simulink model "MultirotorSimFSFBTranslationOnly"  (R2018b)
settings: Solver=VariableStepAuto  StartTime=0.0  StopTime=Simulation.T_END  MaxStep=Simulation.TS_MAX  RelTol=1e-3  EnableMultiTasking=on
PreLoadFcn:
  | % InitializeParameters;
undefined symbols (not defined in the file): Aero, Initial, K, Uav, Wind
libraries: QuaternionLibrary x12
settings Model: Creator=jban039  LastModifiedBy=jban039
settings DataIOCC: Decimation=10  ExternalInput=getinputstruct(op)  InitialState=getstatestruct(op)  SaveFormat=StructureWithTime  SignalLogging=off  ReturnWorkspaceOutputs=on  OutputTimes=Simulation.T_OUT
settings OptimizationCC: LifeSpan=inf
settings DebuggingCC: ReadBeforeWriteMsg=DisableAll  WriteAfterWriteMsg=DisableAll  WriteAfterReadMsg=DisableAll  MultiTaskDSMMsg=none  UnconnectedLineMsg=none  AllowSymbolicDim=off  SFUnexpectedBacktrackingDiag=warning  SFNoUnconditionalDefaultTransitionDiag=warning  SFExecutionAtInitializationDiag=none
settings ModelReferenceCC: UpdateModelReferenceTargets=IfOutOfDate  ModelReferenceMinAlgLoopOccurrences=on  PropagateSignalLabelsOutOfModel=off
settings SFSimCC: SFSimEcho=off  SimUseLocalCustomCode=off
settings RTWCC: RTWUseLocalCustomCode=off
settings CodeAppCC: StateflowObjectComments=on
settings GRTTargetCC: TargetLangStandard=C89/C90 (ANSI)
settings ConfigComp: CovMetricSettings=dw  CovHtmlReporting=on  CovSaveCumulativeToWorkspaceVar=on  CovSaveSingleToWorkspaceVar=on  CovExternalEMLEnable=off

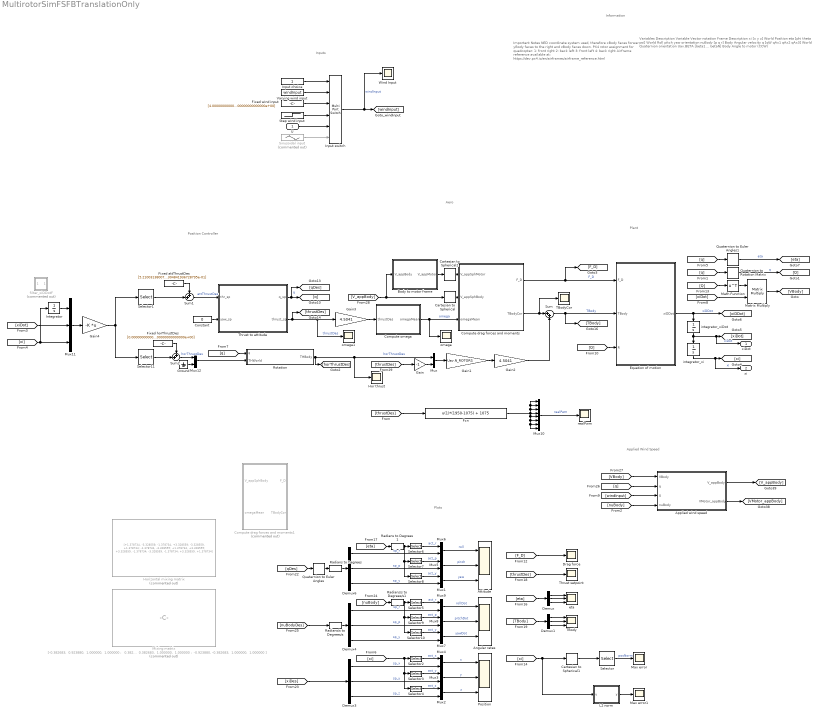
== system MultirotorSimFSFBTranslationOnly ==
  note: Plots
  note: Inputs
  note: Plant
  note: Position Controller
  note: Applied Wind Speed
  note: Important Notes
      |
      | NED coordinate system used, therefore xBody faces forward, yBody faces to the right and zBody faces down.
      | PX4 rotor assignment for quadcopter:
      | 1: front right
      | 2: back left
      | 3: front left
      | 4: back right
      | Airframe reference available at:
      | https://dev.px4.io/en/airframes/airframe_reference.html
  note: Variables Description
      |
      | Variable
      | Vector notation
      | Frame
      | Description
      |
      | xi
      | [x y z]
      | World
      | Position
      |
      | eta
      | [phi theta psi]
      | World
      | Roll pitch yaw orientation
      |
      | nuBody
      | [p q r]
      | Body
      | Angular velocity
      |
      | q
      | [qW qAx1 qAx2 qAx3]
      | World
      | Quaternion orientation
      |
      | Uav.BETA
      | [beta1 ... betaN]
      | Body
      | Angle to motor (CCW)
  note: Information
  note: Aero
  U : Inport  PortDimensions=3
  Angular rates : Scope  NumInputPorts=3
  Applied wind speed : Subsystem
  Attitude : Scope  NumInputPorts=3
  Body to motor frame : MATLAB Function  TreatAsAtomicUnit=on
  Cartesian to Spherical : QuaternionLibrary/Cartesian to Spherical
  Cartesian to Spherical1 : QuaternionLibrary/Cartesian to Spherical
  Cartesian to Spherical2 : QuaternionLibrary/Cartesian to Spherical
  Compute drag forces and moments : MATLAB Function  TreatAsAtomicUnit=on
  Compute drag forces and moments1 : MATLAB Function  Commented=on  TreatAsAtomicUnit=on
  Compute omega : MATLAB Function  TreatAsAtomicUnit=on
  Constant : Constant  Value=0
  Demux{,1,3..4,6} (5 alike) : Demux  Outputs=3
  Drag force : Scope
  Equation of motion : MATLAB Function  TreatAsAtomicUnit=on
  Fcn : Fcn  Expr=u(1)*(1950-1075) + 1075
  Fixed attThrustDes : Constant  Value=[5.210031380070558e-02;0.000000000000000e+00;-5.304841936728795e-01]
  Fixed horThrustDes : Constant  Value=[0.000000000000000e+00;0.000000000000000e+00]
  Fixed wind input : Constant  Value=[4.000000000000000e+00;0.000000000000000e+00;0.000000000000000e+00]
  Gain : Gain  Gain=-1
  Gain1 : Gain  Gain=Uav.N_ROTORS
  Gain2 : Gain  Gain=4.5041
  Gain3 : Gain  Gain=4.5041
  Gain4 : Gain  Gain=-K  Multiplication=Matrix(K*u)
  Ground : Ground
  Hor thrust : Scope
  Horizontal mixing matrix : Constant  Commented=on  Value=|
      | [+1.378734, -3.328559;
      |  -1.378734, +3.328559;
      |  -3.328559, +1.378734;
      |  -1.378734, -3.328559;
      |  +1.378734, +3.328559;
      |  +3.328559, -1.378734;
      |  -3.328559, -1.378734;
      |  +3.328559, +1.378734]
  Input choice : Constant
  Input switch : MultiPortSwitch  Inputs=5
  Integrator : Integrator
  L2 norm : MATLAB Function  TreatAsAtomicUnit=on
  Math Function : Math  Operator=transpose  SaturateOnIntegerOverflow=on
  Matrix Multiply : Product  Multiplication=Matrix(*)
  Max error : Scope
  Max error1 : Scope
  Mixing matrix : Constant  Commented=on  Value=|
      | [-0.382683,  0.923880,  1.000000,  1.000000 ;
      |   0.382683, -0.923880,  1.000000,  1.000000 ;
      |  -0.923880,  0.382683, -1.000000,  1.000000 ;
      |  -0.382683, -0.923880, -1.000000,  1.000000 ;
      |   0.382683,  0.923880, -1.000000,  1.000000 ;
      |   0.923880, -0.382683, -1.000000,  1.000000 ;
      |   0.923880,  0.382683,  1.000000,  1.000000 ;
      |  -0.923880, -0.382683,  1.000000,  1.000000 ]
  Mux{,1..9,12} (11 alike) : Mux  Inputs=2
  Mux10 : Mux  Inputs=8
  Mux11 : Mux  Inputs=3
  Position : Scope  NumInputPorts=3
  Quaternion to Euler Angles : QuaternionLibrary/Quaternion to Euler Angles
  Quaternion to Euler Angles1 : QuaternionLibrary/Quaternion to Euler Angles
  Quaternion to Rotation Matrix : QuaternionLibrary/Quaternion to Rotation Matrix
  "Radians to Degrees " : QuaternionLibrary/Radians to Degrees   SystemSampleTime=-1
  Radians to Degrees 1 : QuaternionLibrary/Radians to Degrees   SystemSampleTime=-1
  Radians/s to Degrees/s : QuaternionLibrary/Radians//s to Degrees//s  SystemSampleTime=-1
  Radians/s to Degrees/s1 : QuaternionLibrary/Radians//s to Degrees//s  SystemSampleTime=-1
  Rotation : Subsystem
  Selector : Selector  InputPortWidth=3  IndexOptions=Index vector (dialog)  Indices=[3]  OutputSizes=1
  Selector1 : Selector  InputPortWidth=5  IndexOptions=Index vector (dialog)  Indices=[3:5]  OutputSizes=1
  Selector10 : Selector  InputPortWidth=3  IndexOptions=Index vector (dialog)  Indices=3  OutputSizes=1
  Selector11 : Selector  InputPortWidth=5  IndexOptions=Index vector (dialog)  Indices=[1 2]  OutputSizes=1
  Selector2 : Selector  InputPortWidth=3  IndexOptions=Index vector (dialog)  Indices=1  OutputSizes=1
  Selector3 : Selector  InputPortWidth=3  IndexOptions=Index vector (dialog)  Indices=2  OutputSizes=1
  Selector4 : Selector  InputPortWidth=3  IndexOptions=Index vector (dialog)  Indices=3  OutputSizes=1
  Selector5 : Selector  InputPortWidth=3  IndexOptions=Index vector (dialog)  Indices=1  OutputSizes=1
  Selector6 : Selector  InputPortWidth=3  IndexOptions=Index vector (dialog)  Indices=1  OutputSizes=1
  Selector7 : Selector  InputPortWidth=3  IndexOptions=Index vector (dialog)  Indices=2  OutputSizes=1
  Selector8 : Selector  InputPortWidth=3  IndexOptions=Index vector (dialog)  Indices=3  OutputSizes=1
  Selector9 : Selector  InputPortWidth=3  IndexOptions=Index vector (dialog)  Indices=2  OutputSizes=1
  Sinusoidal input : Sin  Commented=on  Amplitude=Wind.Ampl  Bias=Wind.Bias  Frequency=Wind.Freq  SampleTime=0
  Step wind input : Step  Time=Wind.StepTime  Before=Wind.StepInit  After=Wind.StepFinal  SampleTime=0
  Sum : Sum  Inputs=|++
  Sum1 : Sum  Inputs=++|
  Sum2 : Sum  Inputs=++|
  TBody : Scope  NumInputPorts=3
  TBodyCor : Scope
  Thrust setpoint : Scope
  Thrust to attitude : MATLAB Function  TreatAsAtomicUnit=on
  Varying wind input : FromWorkspace  VariableName=windInput  SampleTime=0
  Wind Input : Scope
  eta : Scope  NumInputPorts=3
  filter_xiDDotF : Subsystem  Commented=on  mask{PID_FC=5}
      mask prompts: PID_FC "D filter cutoff"
      mask Display: disp('s')
  integrator_xi : Integrator  InitialCondition=Initial.XI  ContinuousStateAttributes='xi'
  integrator_xiDot : Integrator  InitialCondition=Initial.XI_DOT  ContinuousStateAttributes='xiDot'
  omega : Scope
  omega1 : Scope
  realPwm : Scope
  xiDot : Outport
  xi : Outport  Port=2
  wires:
  Sum/1 -> Equation of motion/2(TBody), [TBody]  "TBody"
  Matrix Multiply/1 -> [VBody]
  integrator_xi/1 -> xi/1, [xi]  "xi"
  integrator_xiDot/1 -> xiDot/1, [xiDot], integrator_xi/1  "xiDot"
  Equation of motion/1(xiDDot) -> [xiDDot], integrator_xiDot/1  "xiDDot"
  Quaternion to Euler Angles1/1 -> [eta]  "eta"
  Thrust to attitude/1(q_sp) -> [q], [qDes]  "q"
  [VBody] -> Applied wind speed/1(VBody)
  [q] -> Applied wind speed/2(q)
  [windInput] -> Applied wind speed/3(U)
  Applied wind speed/1(V_appBody) -> [V_appBody]
  Applied wind speed/2(VMotor_appBody) -> [VMotor_appBody]
  [nuBody] -> Applied wind speed/4(nuBody)
  Mux7/1 -> Angular rates/3  "yawDot"
  [nuBody] -> Radians/s to Degrees/s1/1
  Radians/s to Degrees/s1/1 -> Selector5/1, Selector9/1, Selector10/1
  Radians/s to Degrees/s/1 -> Demux4/1
  Mux8/1 -> Angular rates/2  "pitchDot"
  Mux9/1 -> Angular rates/1  "rollDot"
  Selector10/1 -> Mux7/1  "act_y"
  Demux4/2 -> Mux8/2  "sp_p"
  Demux4/1 -> Mux9/2  "sp_r"
  [nuBodyDes] -> Radians/s to Degrees/s/1
  Selector9/1 -> Mux8/1  "act_p"
  Selector5/1 -> Mux9/1  "act_r"
  Demux4/3 -> Mux7/2  "sp_y"
  Mux2/1 -> Position/3  "z"
  [xi] -> Selector2/1, Selector3/1, Selector4/1
  [xiDes] -> Demux3/1
  Mux3/1 -> Position/2  "y"
  Mux4/1 -> Position/1  "x"
  Selector4/1 -> Mux2/1  "act_z"
  Demux3/2 -> Mux3/2  "sp_y"
  Demux3/1 -> Mux4/2  "sp_x"
  Selector3/1 -> Mux3/1  "act_y"
  Selector2/1 -> Mux4/1  "act_x"
  Demux3/3 -> Mux2/2  "sp_z"
  L2 norm/1(y) -> Max error1/1
  [F_D] -> Drag force/1
  Selector/1 -> Max error/1  "posNorm"
  Demux1/1 -> TBody/1
  [TBody] -> Demux1/1
  Demux1/2 -> TBody/2
  Demux1/3 -> TBody/3
  [thrustDes] -> Thrust setpoint/1
  Demux6/3 -> Mux1/2  "sp_y"
  Selector6/1 -> Mux6/1  "act_r"
  Selector7/1 -> Mux5/1  "act_p"
  Quaternion to Euler Angles/1 -> "Radians to Degrees "/1
  Demux6/1 -> Mux6/2  "sp_r"
  Demux6/2 -> Mux5/2  "sp_p"
  Selector8/1 -> Mux1/1  "act_y"
  [qDes] -> Quaternion to Euler Angles/1
  Mux6/1 -> Attitude/1  "roll"
  Mux5/1 -> Attitude/2  "pitch"
  "Radians to Degrees "/1 -> Demux6/1
  Radians to Degrees 1/1 -> Selector8/1, Selector7/1, Selector6/1
  [eta] -> Radians to Degrees 1/1
  Mux1/1 -> Attitude/3  "yaw"
  Demux/3 -> eta/3
  Demux/2 -> eta/2
  Demux/1 -> eta/1
  [eta] -> Demux/1
  [xi] -> Cartesian to Spherical1/1, L2 norm/1(u)
  Sinusoidal input/1 -> Input switch/6
  U/1 -> Input switch/5
  Input choice/1 -> Input switch/1
  Step wind input/1 -> Input switch/4
  Input switch/1 -> [windInput], Wind Input/1  "windInput"
  Fixed wind input/1 -> Input switch/3
  Varying wind input/1 -> Input switch/2
  [Q] -> Equation of motion/3(R)
  [q] -> Quaternion to Euler Angles1/1
  [q] -> Quaternion to Rotation Matrix/1
  Quaternion to Rotation Matrix/1 -> [Q]  "q"
  Math Function/1 -> Matrix Multiply/1
  [xiDot] -> Matrix Multiply/2
  [Q] -> Math Function/1
  [V_appBody] -> Cartesian to Spherical/1, Body to motor frame/1(V_appBody)
  Cartesian to Spherical/1 -> Compute drag forces and moments/2(V_appSphBody)
  Compute omega/1(omegaMean) -> Compute drag forces and moments/3(omegaMean), omega/1  "omega"
  Rotation/1(THBody) -> [horThrustDes], Mux/1, Hor thrust/1  "horThrustDes"
  [thrustDes] -> Gain/1
  Compute drag forces and moments/1(F_D) -> [F_D], Equation of motion/1(F_D)  "F_D"
  Compute drag forces and moments/2(TBodyCor) -> TBodyCor/1, Sum/1
  Mux/1 -> Gain1/1
  Gain/1 -> Mux/2
  Gain2/1 -> Sum/2
  Gain3/1 -> Compute omega/1(thrustDes)
  [thrustDes] -> Fcn/1
  Mux10/1 -> realPwm/1  "realPwm"
  Fcn/1 -> Mux10/8, Mux10/7, Mux10/6, Mux10/5, Mux10/1, Mux10/2, Mux10/3, Mux10/4
  Thrust to attitude/2(thrust_sp) -> omega1/1, Gain3/1, [thrustDes]  "thrustDes"
  Fixed horThrustDes/1 -> Sum2/1
  Cartesian to Spherical1/1 -> Selector/1
  Gain1/1 -> Gain2/1
  Body to motor frame/1(V_appMotor) -> Cartesian to Spherical2/1
  Cartesian to Spherical2/1 -> Compute drag forces and moments/1(V_appSphMotor)
  Constant/1 -> Thrust to attitude/2(yaw_sp)
  Sum1/1 -> Thrust to attitude/1(thr_sp)  "attThrustDes"
  Fixed attThrustDes/1 -> Sum1/1
  Selector1/1 -> Sum1/2
  Selector11/1 -> Sum2/2
  [xiDot] -> Mux11/2
  [xi] -> Mux11/3, Integrator/1
  Mux11/1 -> Gain4/1
  Gain4/1 -> Selector1/1, Selector11/1
  Integrator/1 -> Mux11/1
  Sum2/1 -> Mux12/1  "horThrustDes"
  Ground/1 -> Mux12/2
  Mux12/1 -> Rotation/2(THWorld)
  [q] -> Rotation/1(q)

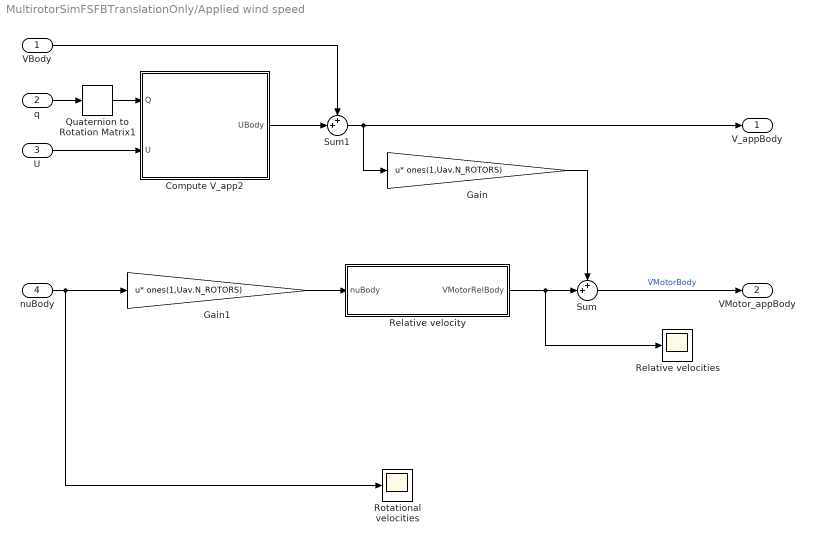
== system MultirotorSimFSFBTranslationOnly/Applied wind speed ==
  VBody : Inport  Unit=m/s
  q : Inport  Port=2
  U : Inport  Port=3  Unit=m/s
  nuBody : Inport  Port=4  Unit=rad/s
  Compute V_app2 : MATLAB Function  TreatAsAtomicUnit=on
  Gain : Gain  Gain=ones(1,Uav.N_ROTORS)  Multiplication=Matrix(u*K)
  Gain1 : Gain  Gain=ones(1,Uav.N_ROTORS)  Multiplication=Matrix(u*K)
  Quaternion to Rotation Matrix1 : QuaternionLibrary/Quaternion to Rotation Matrix
  Relative velocities : Scope
  Relative velocity : MATLAB Function  TreatAsAtomicUnit=on
  Rotational velocities : Scope
  Sum : Sum  Inputs=++|
  Sum1 : Sum  Inputs=++|
  V_appBody : Outport  Unit=m/s
  VMotor_appBody : Outport  Port=2  Unit=m/s  PortDimensions=[3,Uav.N_ROTORS]
  wires:
  U/1 -> Compute V_app2/2(U)
  Sum/1 -> VMotor_appBody/1  "VMotorBody"
  Quaternion to Rotation Matrix1/1 -> Compute V_app2/1(Q)
  nuBody/1 -> Gain1/1, Rotational velocities/1
  Gain/1 -> Sum/1
  VBody/1 -> Sum1/1
  q/1 -> Quaternion to Rotation Matrix1/1
  Relative velocity/1(VMotorRelBody) -> Relative velocities/1, Sum/2
  Compute V_app2/1(UBody) -> Sum1/2
  Sum1/1 -> Gain/1, V_appBody/1
  Gain1/1 -> Relative velocity/1(nuBody)

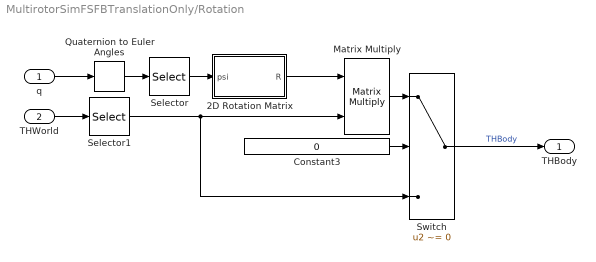
== system MultirotorSimFSFBTranslationOnly/Rotation ==
  q : Inport
  THWorld : Inport  Port=2
  2D Rotation Matrix : Subsystem
  Constant3 : Constant  Value=0
  Matrix Multiply : Product  Multiplication=Matrix(*)
  Quaternion to Euler Angles : QuaternionLibrary/Quaternion to Euler Angles
  Selector : Selector  InputPortWidth=3  IndexOptions=Index vector (dialog)  Indices=3  OutputSizes=1
  Selector1 : Selector  InputPortWidth=3  IndexOptions=Index vector (dialog)  Indices=[1 2]  OutputSizes=1
  Switch : Switch  Criteria=u2 ~= 0
  THBody : Outport
  wires:
  Selector1/1 -> Matrix Multiply/2, Switch/3
  Constant3/1 -> Switch/2
  Selector/1 -> 2D Rotation Matrix/1(psi)
  Quaternion to Euler Angles/1 -> Selector/1
  2D Rotation Matrix/1(R) -> Matrix Multiply/1
  Switch/1 -> THBody/1  "THBody"
  Matrix Multiply/1 -> Switch/1
  THWorld/1 -> Selector1/1
  q/1 -> Quaternion to Euler Angles/1

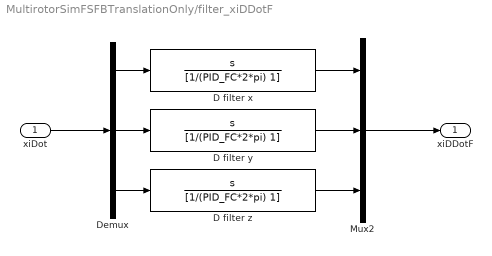
== system MultirotorSimFSFBTranslationOnly/filter_xiDDotF ==
  xiDot : Inport  Unit=m/s
  D filter x : TransferFcn  Numerator=[1 0]  Denominator=[1/(PID_FC*2*pi) 1]  ContinuousStateAttributes='velPID_D_x'
  D filter y : TransferFcn  Numerator=[1 0]  Denominator=[1/(PID_FC*2*pi) 1]  ContinuousStateAttributes='velPID_D_y'
  D filter z : TransferFcn  Numerator=[1 0]  Denominator=[1/(PID_FC*2*pi) 1]  ContinuousStateAttributes='velPID_D_z'
  Demux : Demux  Outputs=3
  Mux2 : Mux  Inputs=3
  xiDDotF : Outport  Unit=m/s^2
  wires:
  Mux2/1 -> xiDDotF/1
  Demux/3 -> D filter z/1
  Demux/1 -> D filter x/1
  D filter z/1 -> Mux2/3
  xiDot/1 -> Demux/1
  D filter y/1 -> Mux2/2
  Demux/2 -> D filter y/1
  D filter x/1 -> Mux2/1

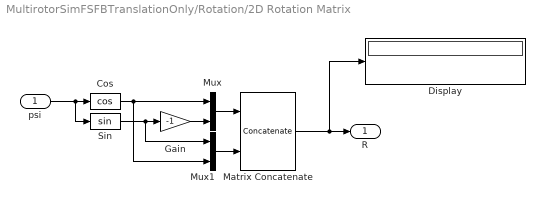
== system MultirotorSimFSFBTranslationOnly/Rotation/2D Rotation Matrix ==
  psi : Inport
  Cos : Trigonometry  Operator=cos
  Display : Display
  Gain : Gain  Gain=-1
  Matrix Concatenate : Concatenate  Mode=Multidimensional array  ConcatenateDimension=2
  Mux : Mux  Inputs=2
  Mux1 : Mux  Inputs=2
  Sin : Trigonometry
  R : Outport
  wires:
  psi/1 -> Cos/1, Sin/1
  Matrix Concatenate/1 -> R/1, Display/1
  Mux1/1 -> Matrix Concatenate/2
  Gain/1 -> Mux/2
  Mux/1 -> Matrix Concatenate/1
  Sin/1 -> Gain/1, Mux1/1
  Cos/1 -> Mux/1, Mux1/2

== matlab function MultirotorSimFSFBTranslationOnly/Body to motor frame ==
  data: V_appBody input; V_appMotor output; Uav parameter
function V_appMotor = BodyToMotor( V_appBody, Uav )
%#codegen
    V_appMotor = [Uav.GAMMA';Uav.GAMMA';Uav.GAMMA'] .* 0;
    for i = 1:Uav.N_ROTORS
        V_appMotor(:,i) = Uav.R_MOTOR_TO_BODY(:,:,i)' * V_appBody;
    end
end

== matlab function MultirotorSimFSFBTranslationOnly/Compute omega ==
  data: thrustDes input; omegaMean output; Uav parameter; Aero parameter
function omegaMean = CalcOmega( thrustDes, Uav, Aero)
%#codegen
    thrustDesMotor = thrustDes ./ cos(Uav.ZETA);
    Cz2 = dot( Aero.Cz2.coefs, [0, 1]);
    omegaMean = sqrt( thrustDesMotor .* 2 ./ ( Uav.RHO_AIR .* Cz2 .* Uav.D_PROP^2 .* Uav.A_PROP ) );
end

== matlab function MultirotorSimFSFBTranslationOnly/Compute drag forces and moments1 ==
  data: V_appSphBody input; omegaMean input; F_D output; Uav parameter; Aero parameter; TBodyCor output
function [F_D, TBodyCor] = ComputeAero( V_appSphBody, omegaMean, Uav, Aero )
%#codegen
    % Body aerodynamic forces
    beta  = V_appSphBody(1);
    alpha = V_appSphBody(2);
    U     = V_appSphBody(3);

    Cz1 = dot( Aero.Cz1.coefs, [sin(alpha), 1] );
    Cx1 = dot( Aero.Cx1.coefs, [cos(alpha), cos(3*alpha), cos(7*alpha)] );
    faero_z = -0.5 .* Uav.RHO_AIR .* U^2 .* Cz1 * Uav.A_UAV;
    faero_x = -0.5 .* Uav.RHO_AIR .* U^2 .* Cx1 * Uav.A_UAV;
    F_D = [faero_x*cos(beta); faero_x*sin(beta); faero_z];

    % Rotor aerodynamic forces
    lambda = omegaMean * Uav.D_PROP / ( 2 * U );
    p = Aero.Cx2.coefs;
    Cx2 = p(1) * ( 1 - exp(-p(2).*lambda) ) .* cos(alpha) + ...
          p(3) * ( 1 - exp(-p(4).*lambda) ) .* cos(3*alpha);
    Tx    = -0.5 .* Uav.RHO_AIR .* (Cx2)' .* U .* omegaMean' .* Uav.D_PROP .* Uav.A_PROP;
    TBodyHor = [ Tx.*cos(beta); Tx.*sin(beta); 0 ] .* Uav.N_ROTORS;
    
    TBodyIndividual   = zeros(3,Uav.N_ROTORS);
    for i = 1:Uav.N_ROTORS
        p = Aero.Cz3.coefs;
        Cz3 = p(1) * sin(alpha) + p(2) * ( 1 - exp(-p(3).*lambda) ) .* sin(3*alpha) + ...
            p(4);
        TzCor = - 0.5 .* Uav.RHO_AIR .* (Cz3)' .* U .*  omegaMean' .* Uav.D_PROP .* Uav.A_PROP; % Rotor thrust correction
        TMotorIndividual = [ 0; 0; TzCor ];

        % Motor force/torque vectors in body frame
        TBodyIndividual(:,i) = Uav.R_MOTOR_TO_BODY(:,:,i) * ...
            TMotorIndividual;
    end
    
    TBodyCor = sum(TBodyIndividual, 2) + TBodyHor;
end

== matlab function MultirotorSimFSFBTranslationOnly/Applied wind speed/Relative velocity ==
  data: nuBody input; Uav parameter; VMotorRelBody output
function VMotorRelBody = relativeMotorVelocity( nuBody , Uav )
%#codegen
    VMotorRelBody = cross( nuBody, Uav.L_VEC );
end

== matlab function MultirotorSimFSFBTranslationOnly/Applied wind speed/Compute V_app2 ==
  data: Q input; UBody output; U input size=3
function UBody = computeUBody(Q, U)
%#codegen

% Rotation matrix from Wind frame to Inertial frame
% Wind frame SEU, inertial frame NED
R_U = [1,  0, 0;
       0, -1, 0;
       0,  0, 1];
   
UBody = Q' * R_U * U;

== matlab function MultirotorSimFSFBTranslationOnly/Equation of motion ==
  data: F_D input size=3; TBody input size=3; R input; Uav parameter; xiDDot output
function xiDDot = QuadrotorTranslationModel( F_D, TBody, R, Uav )
%#codegen

%% Moments and Forces
xiDDot = (1/Uav.M)*(Uav.G + R*TBody + R*F_D);

end

== matlab function MultirotorSimFSFBTranslationOnly/Thrust to attitude ==
  data: thr_sp input size=3; q_sp output; yaw_sp input; thrust_sp output
function [q_sp, thrust_sp] = thrustToAttitude( thr_sp, yaw_sp )
%#codegen
    yaw_body = yaw_sp;
    body_z = -thr_sp./norm(thr_sp);
    
    y_C = [ -sin(yaw_body); cos(yaw_body); 0 ];
    
    body_x = zeros(3,1);
    if body_z(3) > 0.000001
        body_x = cross( y_C, body_z );
        if ( body_z(3) < 0 )
            body_x = -body_x;
        end
        
        body_x = body_x ./ norm(body_x);
    else
        body_x(3) = 1;
    end
    
    body_y = cross( body_z, body_x );
    
    R_sp = [ body_x, body_y, body_z ];
    
    q_sp = from_dcm( R_sp );
    
    thrust_sp = norm( thr_sp );
end

function data  = from_dcm( dcm )
% FROM_DCM Convert DCM to quaternion
% From https://github.com/PX4/Firmware/blob/master/src/lib/mathlib/math/Quaternion.hpp
    data = zeros(4,1);
    tr = dcm(1,1) + dcm(2,2) + dcm(3,3);
    if (tr > 0.0)
        s = sqrt(tr + 1.0);
        data(1) = s * 0.5;
        s = 0.5 / s;
        data(2) = (dcm(3,2) - dcm(2,3) ) * s;
        data(3) = (dcm(1,3) - dcm(3,1) ) * s;
        data(4) = (dcm(2,1) - dcm(1,2) ) * s;
    else
        % Find maximum diagonal element in dcm
        % store index in dcm_i
        dcm_i = 1;
        for i = 2:3 % (int i = 1; i < 3; i++)
            if ( dcm(i,i) > dcm(dcm_i,dcm_i) )
                dcm_i = i;
            end
        end
        dcm_j = rem( ( (dcm_i-1) + 1), 3) + 1;
        dcm_k = rem( ( (dcm_i-1) + 2), 3) + 1;
        s = sqrt( (dcm(dcm_i, dcm_i) - dcm(dcm_j, dcm_j) - ...
            dcm(dcm_k,dcm_k)) + 1.0 );
        data(dcm_i + 1) = s * 0.5;
        s = 0.5 / s;
        data(dcm_j + 1) = ( dcm(dcm_i,dcm_j) + dcm(dcm_j,dcm_i) ) * s;
        data(dcm_k + 1) = ( dcm(dcm_k,dcm_i) + dcm(dcm_i,dcm_k) ) * s;
        data(1) = ( dcm(dcm_k,dcm_j) - dcm(dcm_j,dcm_k) ) * s;
    end
end

== matlab function MultirotorSimFSFBTranslationOnly/Compute drag forces and moments ==
  data: V_appSphMotor input; V_appSphBody input; omegaMean input; F_D output; Uav parameter; Aero parameter; TBodyCor output
function [F_D, TBodyCor] = ComputeAero( V_appSphMotor, V_appSphBody, omegaMean, Uav, Aero )
%#codegen
    % Body aerodynamic forces
    betaBody  = V_appSphBody(1);
    alphaBody = V_appSphBody(2);
    U         = V_appSphBody(3);

    Cz1 = dot( Aero.Cz1.coefs, [sin(alphaBody), 1] );
    Cx1 = dot( Aero.Cx1.coefs, [cos(alphaBody), cos(3*alphaBody), cos(7*alphaBody)] );
    faero_z = -0.5 .* Uav.RHO_AIR .* U^2 .* Cz1 * Uav.A_UAV;
    faero_x = -0.5 .* Uav.RHO_AIR .* U^2 .* Cx1 * Uav.A_UAV;
    F_D = [faero_x*cos(betaBody); faero_x*sin(betaBody); faero_z];

    % Rotor aerodynamic forces
    beta  = V_appSphMotor(1,:);
    alpha = V_appSphMotor(2,:);
    lambda = omegaMean * Uav.D_PROP / ( 2 * U );

    p = Aero.Cx2.coefs;
    Cx2 = p(1) * ( 1 - exp(-p(2).*lambda) ) .* cos(alpha) + ...
          p(3) * ( 1 - exp(-p(4).*lambda) ) .* cos(3.*alpha);
    Tx    = -0.5 .* Uav.RHO_AIR .* (Cx2) .* U .* omegaMean' .* Uav.D_PROP .* Uav.A_PROP;

    p = Aero.Cz3.coefs;
    Cz3 = p(1) * sin(alpha) + p(2) * ( 1 - exp(-p(3).*lambda) ) .* sin(3.*alpha) + p(4);
    TzCor = - 0.5 .* Uav.RHO_AIR .* Cz3 .* U .* omegaMean' .* Uav.D_PROP .* Uav.A_PROP; % Rotor thrust correction

    TMotorIndividual = [  Tx.*cos(beta); Tx.*sin(beta); TzCor ];
    TBodyIndividual = TMotorIndividual .* 0;
    for i = 1:Uav.N_ROTORS
        % Motor force/torque vectors in body frame
        TBodyIndividual(:,i) = Uav.R_MOTOR_TO_BODY(:,:,i) * ...
            TMotorIndividual(:,i);
    end
    
    TBodyCor = sum(TBodyIndividual, 2);
end

== matlab function MultirotorSimFSFBTranslationOnly/L2 norm ==
  data: u input; y output
function y = l2norm( u )
    y = sqrt( dot(u, u) );
end
